simulink model "eVTOL_PX4_2023b"  (R2024b)
settings: Solver=ode4  StartTime=0  StopTime=inf  FixedStep=0.01  RelTol=1e-3
values from neighbouring files (symbols this model uses):
  aDl =     [initdata.mat]
  aDr =     [initdata.mat]
  aDyn =     [initdata.mat]
  Airport = init_airport('PHNL')    [initdata_HIL_eVTOL.m]
  aLat =     [initdata.mat]
  aLon =     [initdata.mat]
  D = Prop.D    [EOM_dt_MC.m]    (also in EOM_get_alf_dt_de_prop_evtol.m = CD * QS)
  dt0 = X(2)    [EOM_get_alf_dt_de_prop_evtol.m]    (also in initdata.mat = 0.258252593971; initdata_HIL_eVTOL.m = EOM_dt_MC)
  EAS0 = TAS0 / EAS2TAS    [initdata_HIL_eVTOL.m]
  FCS = init_FCS    [initdata_HIL_eVTOL.m]
  General = init_layoutdata    [EOM_dt_MC.m]    (also in build_optimized_CA.m; initdata.mat = ; initdata_HIL_eVTOL.m)
  h0 = Con(1)    [EOM_get_alf_dt_de_prop_evtol.m]    (also in initdata.mat = 450; initdata_HIL_eVTOL.m = 50)
  mass = Con(3)    [EOM_get_alf_dt_de_prop_evtol.m]    (also in initdata.mat = 2255.54; initdata_HIL_eVTOL.m = 7)
  Motor = init_motor_evtol    [EOM_dt_MC.m]    (also in initdata.mat = []; initdata_HIL_eVTOL.m)
  Prop = init_propeller_evtol_new    [EOM_dt_MC.m]    (also in initdata_HIL_eVTOL.m)
  R2D = 180/pi    (= 57.2957795131)    [EOM_get_alf_dt_de_prop_evtol.m]    (also in init_FCS.m; init_aerodata_evtol.m; init_airport.m; initdata.mat)
  SAMPLE_TIME = 0.01    [initdata_HIL_eVTOL.m]
  theta0 = -0.0510981441662    [initdata.mat]
undefined symbols (not defined in the file or in its folder): A1, aDa, aDe, aero, asbhl20env, B1, C1, de0, Earth, Environment, INIT_Data, InitData, Kd, Kp, magnitude, Newton, pProp, Raphson, Tc, WGS84
libraries: simulink_extras x63, vrlib x48, sharedtransform x28, simulink x22, slpidlib x20, sharedutil x20, matrix_library x18, aerolibwindfilters x12, aerolibobsolete x8, aerolibasang x8, aerolibatmos2 x6, aerolibfltsims x6
(part 2 of 17)

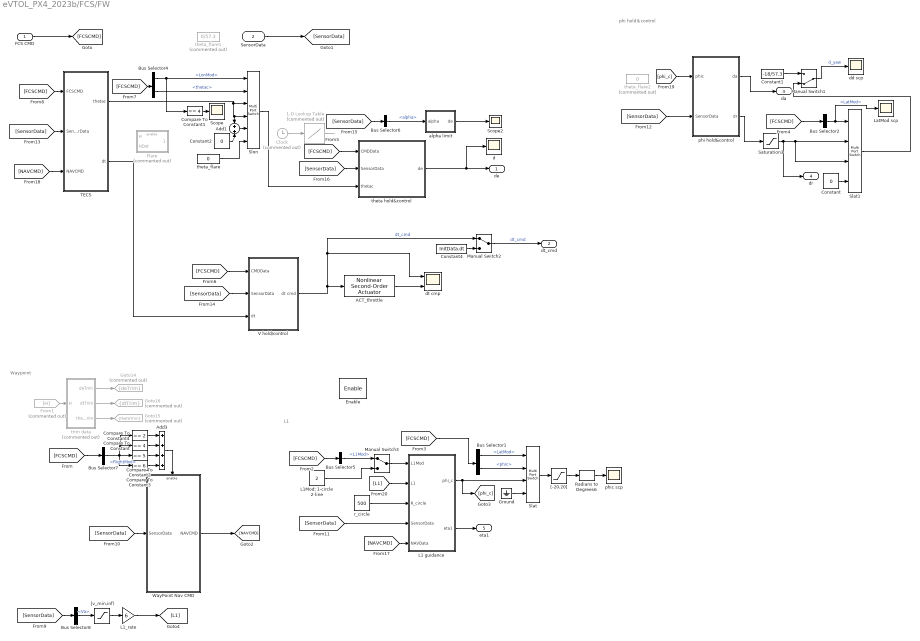
== system eVTOL_PX4_2023b/FCS/FW ==
  note: phi hold＆control
  note: L1
  note: Waypoint
  FCS CMD : Inport
  SensorData : Inport  Port=2
  Enable : EnablePort  StatesWhenEnabling=reset
  1-D Lookup Table : Lookup_n-D  Commented=on  NumberOfTableDimensions=1  BreakpointsForDimension1=[0,4,13,1e3]  Table=[-90,-90,0,0]./57.3  InternalRulePriority=Speed  RndMeth=Simplest
  ACT_throttle : aerolibactuator/Nonlinear Second-Order Actuator  wn_fin=50  z_fin=0.8  fin_max=FCS.dt_max  fin_min=FCS.dt_min  fin_maxrate=FCS.dt_rate  fin_act_0=InitData.dt  fin_act_vel=0
  Add1 : Sum  Inputs=+|+
  Add3 : Sum  Inputs=++++
  Bus Selector1 : BusSelector  OutputSignals=LatMod,phic
  Bus Selector2 : BusSelector  OutputSignals=LatMod
  Bus Selector4 : BusSelector  OutputSignals=LonMod,thetac
  Bus Selector5 : BusSelector  OutputSignals=L1Mod
  Bus Selector6 : BusSelector  OutputSignals=alpha
  Bus Selector7 : BusSelector  OutputSignals=FlightMod
  Bus Selector8 : BusSelector  OutputSignals=Va
  Clock : Clock  Commented=on
  Compare To Constant : simulink/Logic and Bit Operations/Compare To Constant  relop===  const=4  OutDataTypeStr=boolean
  Compare To Constant1 : simulink/Logic and Bit Operations/Compare To Constant  relop===  const=4  OutDataTypeStr=uint8  ZeroCross=off
  Compare To Constant2 : simulink/Logic and Bit Operations/Compare To Constant  relop===  const=5  OutDataTypeStr=boolean
  Compare To Constant3 : simulink/Logic and Bit Operations/Compare To Constant  relop===  const=6  OutDataTypeStr=boolean
  Compare To Constant4 : simulink/Logic and Bit Operations/Compare To Constant  relop===  const=2  OutDataTypeStr=boolean
  Constant : Constant  Value=0
  Constant1 : Constant  Value=-18/57.3
  Constant2 : Constant  Value=0
  Constant4 : Constant  Value=InitData.dt
  Flare : Subsystem  Commented=on
  From1 : From  Commented=on  GotoTag=H
      settings: CloseFcn=tagdialog Close
  Goto14 : Goto  Commented=on  GotoTag=deTrim  TagVisibility=scoped
  Goto15 : Goto  Commented=on  GotoTag=thetaTrim  TagVisibility=scoped
  Goto16 : Goto  Commented=on  GotoTag=dtTrim  TagVisibility=scoped
  Ground : Ground
  L1 guidance : Subsystem
  L1Mod: 1-circle 2-line : Constant  Value=2
  L1_rate : Gain  Gain=6
  LatMod scp : Scope
  Manual Switch1 : ManualSwitch  CurrentSetting=0
  Manual Switch2 : ManualSwitch
  Manual Switch3 : ManualSwitch
  Radians to Degrees6 : simulink_extras/Transformations/Radians to Degrees
  Saturation3 : Saturate  UpperLimit=0.3  LowerLimit=-0.3
  Scope : Scope
  Scope2 : Scope
  Slat : MultiPortSwitch  SaturateOnIntegerOverflow=off  InputSameDT=off
  Slat1 : MultiPortSwitch  SaturateOnIntegerOverflow=off  InputSameDT=off
  Slon : MultiPortSwitch  Inputs=5  SaturateOnIntegerOverflow=off  InputSameDT=off
  TECS : Subsystem
  V hold/control : Subsystem
  WayPoint Nav CMD : Subsystem
  "[-20,20]" : Saturate  UpperLimit=20*pi/180  LowerLimit=-20*pi/180
  "[v_min,inf)" : Saturate  UpperLimit=inf  LowerLimit=FCS.V_min
  alpha limit : Subsystem
  d : Scope
  dd scp : Scope
  dt cmp : Scope  NumInputPorts=2
  phi hold&control : Subsystem
  phic scp : Scope
  r_circle : Constant  Value=500
  theta hold&control : Subsystem
  theta_flare : Constant  Value=0
  theta_flare1 : Constant  Commented=on  Value=0/57.3
  theta_flare2 : Constant  Commented=on  Value=0
  trim data : Subsystem  Commented=on
  de : Outport
  dt_cmd : Outport  Port=2
  da : Outport  Port=3
  dr : Outport  Port=4
  eta1 : Outport  Port=5
  wires:
  Compare To Constant4/1 -> Add3/1
  Bus Selector1/1 -> Slat/1  "<LatMod>"
  trim data/1(deTrim) -> Goto14/1
  WayPoint Nav CMD/1(NAVCMD) -> [NAVCMD]
  L1 guidance/2(eta1) -> eta1/1
  Slat/1 -> "[-20,20]"/1
  "[-20,20]"/1 -> Radians to Degrees6/1
  Add3/1 -> WayPoint Nav CMD/Enable
  r_circle/1 -> L1 guidance/3(R_circle)
  alpha limit/1(de) -> Scope2/1
  Ground/1 -> Slat/4
  V hold/control/1(dt cmd) -> Manual Switch2/1, dt cmp/1, ACT_throttle/1  "dt_cmd"
  L1Mod: 1-circle 2-line/1 -> Manual Switch3/2
  Constant4/1 -> Manual Switch2/2
  trim data/3(thetaTrim) -> Goto15/1
  ACT_throttle/1 -> dt cmp/2
  SensorData/1 -> [SensorData]
  Slat1/1 -> Manual Switch1/2
  Manual Switch1/1 -> dd scp/1  "d_yaw"
  Add1/1 -> Slon/5
  theta_flare/1 -> Slon/6
  Bus Selector2/1 -> LatMod scp/1, Slat1/1  "<LatMod>"
  Bus Selector5/1 -> Manual Switch3/1  "<L1Mod>"
  Bus Selector6/1 -> alpha limit/1(alpha)  "<alpha>"
  Bus Selector7/1 -> Compare To Constant3/1, Compare To Constant4/1, Compare To Constant/1, Compare To Constant2/1  "<FlightMod>"
  "[v_min,inf)"/1 -> L1_rate/1
  Clock/1 -> 1-D Lookup Table/1
  TECS/1(thetac) -> Add1/1, Slon/4, Slon/3
  Saturation3/1 -> dr/1, Slat1/3, Slat1/2
  Slon/1 -> theta hold&control/3(thetac)
  Bus Selector4/1 -> Compare To Constant1/1, Slon/1  "<LonMod>"
  1-D Lookup Table/1 -> ?
  TECS/2(dt) -> V hold/control/3(dt)
  Radians to Degrees6/1 -> phic scp/1
  Bus Selector4/2 -> Slon/2  "<thetac>"
  Bus Selector8/1 -> "[v_min,inf)"/1  "<Va>"
  From1/1 -> trim data/1(H)
  Manual Switch3/1 -> L1 guidance/1(L1Mod)
  phi hold&control/2(dr) -> Saturation3/1
  FCS CMD/1 -> [FCSCMD]
  Compare To Constant2/1 -> Add3/3
  Manual Switch2/1 -> dt_cmd/1  "dt_cmd"
  Constant1/1 -> Manual Switch1/1
  Compare To Constant3/1 -> Add3/4
  trim data/2(dtTrim) -> Goto16/1
  Compare To Constant/1 -> Add3/2
  Bus Selector1/2 -> Slat/2  "<phic>"
  Constant2/1 -> Add1/2
  Constant/1 -> Slat1/4
  Compare To Constant1/1 -> Scope/1
  L1 guidance/1(phi_c) -> [phi_c], Slat/3
  theta hold&control/1(de) -> d/1, de/1
  phi hold&control/1(da) -> da/1
  [FCSCMD] -> Bus Selector7/1
  [FCSCMD] -> Bus Selector5/1
  [FCSCMD] -> Bus Selector1/1
  [FCSCMD] -> Bus Selector2/1
  [FCSCMD] -> theta hold&control/1(CMDData)
  [FCSCMD] -> V hold/control/1(CMDData)
  [FCSCMD] -> Bus Selector4/1
  [FCSCMD] -> TECS/1(FCSCMD)
  [SensorData] -> Bus Selector8/1
  [SensorData] -> WayPoint Nav CMD/1(SensorData)
  [SensorData] -> L1 guidance/4(SensorData)
  [SensorData] -> phi hold&control/2(SensorData)
  [SensorData] -> TECS/2(SensorData)
  [SensorData] -> V hold/control/2(SensorData)
  [SensorData] -> Bus Selector6/1
  [SensorData] -> theta hold&control/2(SensorData)
  [NAVCMD] -> L1 guidance/5(NAVData)
  [NAVCMD] -> TECS/3(NAVCMD)
  [phi_c] -> phi hold&control/1(phic)
  L1_rate/1 -> [L1]
  [L1] -> L1 guidance/2(L1)

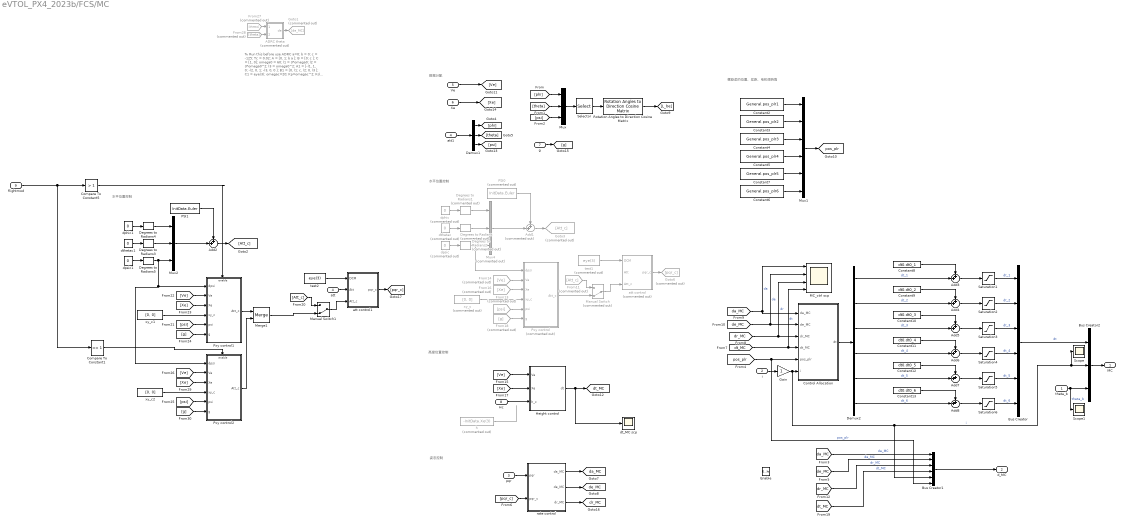
== system eVTOL_PX4_2023b/FCS/MC ==
  note: 数据分配
  note: 螺旋桨的位置、桨距、电机倾转角
  note: 姿态控制
  note: 高度位置控制
  note: 水平位置控制
  note: % Run this before use ADRC
      | a=0;
      | b = 0;
      | c = -125;
      | Tc = 0.02;
      | A = [0, 1; b a ];
      | B = [0; c ];
      | C = [1, 0];
      | omega0 = 60;
      | l1 = 3*omega0;
      | l2 = 3*omega0^2;
      | l3 = omega0^2;
      | A1 = [-l1,  1,  0; -l2,  0,  1; -l3,  0,  0 ];
      | B1 = [0,  l1; c,  l2; 0,  l3 ];
      | C1 = eye(3);
      | omegac=20;
      | Kp=omegac^2;
      | Kd = 2*omegac;
  note: 水平位置控制
  theta_b : Inport
  i : Inport  Port=2
  pqr : Inport  Port=3
  att : Inport  Port=4
  Ve : Inport  Port=5
  Xe : Inport  Port=6
  g : Inport  Port=7
  Hc : Inport  Port=8
  flightmod : Inport  Port=9
  Enable : EnablePort  StatesWhenEnabling=reset
  ADRC theta : Subsystem  Commented=on
  Add1 : Sum  Commented=on  Inputs=++|
  Add{2..8} (7 alike) : Sum  Inputs=++|
  Bus Creator : BusCreator  Inputs=6
  Bus Creator1 : BusCreator  Inputs=6
  Bus Creator2 : BusCreator  Inputs=3
  Compare To Constant1 : simulink/Logic and Bit Operations/Compare To Constant  relop===  const=1  OutDataTypeStr=boolean
  Compare To Constant5 : simulink/Logic and Bit Operations/Compare To Constant  relop=>  const=1  OutDataTypeStr=boolean
  Constant10 : Constant  Value=dt0.dt0_3
  Constant11 : Constant  Value=dt0.dt0_4
  Constant12 : Constant  Value=dt0.dt0_5
  Constant13 : Constant  Value=dt0.dt0_6
  Constant2 : Constant  Value=General.pos_plr1
  Constant3 : Constant  Value=General.pos_plr2
  Constant4 : Constant  Value=General.pos_plr3
  Constant5 : Constant  Value=General.pos_plr4
  Constant6 : Constant  Value=General.pos_plr6
  Constant7 : Constant  Value=General.pos_plr5
  Constant8 : Constant  Value=dt0.dt0_1
  Constant9 : Constant  Value=dt0.dt0_2
  Control Allocation : MATLAB Function  TreatAsAtomicUnit=on
  Degrees to Radians : simulink_extras/Transformations/Degrees to Radians  Commented=on
  Degrees to Radians1 : simulink_extras/Transformations/Degrees to Radians  Commented=on
  Degrees to Radians2 : simulink_extras/Transformations/Degrees to Radians  Commented=on
  Degrees to Radians3 : simulink_extras/Transformations/Degrees to Radians
  Degrees to Radians4 : simulink_extras/Transformations/Degrees to Radians
  Degrees to Radians5 : simulink_extras/Transformations/Degrees to Radians
  Demux1 : Demux  Outputs=3
  Demux2 : Demux  Outputs=6
  From11 : From  Commented=on  GotoTag=Att_c
  From13 : From  Commented=on  GotoTag=psi
  From14 : From  Commented=on  GotoTag=Ve
  From16 : From  Commented=on  GotoTag=Xe
  From18 : From  Commented=on  GotoTag=g
  From27 : From  Commented=on  GotoTag=thetac
  From28 : From  Commented=on  GotoTag=theta
  Gain : Gain
  Goto1 : Goto  Commented=on  GotoTag=de_MC
  Goto3 : Goto  Commented=on  GotoTag=Att_c
  Goto6 : Goto  Commented=on  GotoTag=pqr_c
  Height control : Subsystem
  MC_ctrl scp : Scope  NumInputPorts=4
  Manual Switch : ManualSwitch  Commented=on  CurrentSetting=0
  Manual Switch1 : ManualSwitch  CurrentSetting=0
  Merge1 : Merge
  Mux : Mux  Inputs=3
  Mux1 : Mux  Inputs=6
  Mux2 : Mux  Inputs=3
  Mux4 : Mux  Commented=on  Inputs=3
  PSI0 : Constant  Commented=on  Value=InitData.Euler
  PSI1 : Constant  Value=InitData.Euler
  Pxy control : Subsystem  Commented=on
  Pxy control1 : Subsystem
  Pxy control2 : Subsystem
  Rotation Angles to Direction Cosine Matrix : sharedtransform/Rotation Angles to Direction Cosine Matrix  rotationOrder=ZYX  aMode=aMode
  Saturation{1..6} (6 alike) : Saturate  UpperLimit=1  LowerLimit=0
  Scope : Scope
  Scope1 : Scope
  Selector : Selector  InputPortWidth=3  IndexOptions=Index vector (dialog)  Indices=[3,2,1]  OutputSizes=1
  att control : Subsystem  Commented=on
  att control1 : Subsystem
  att1 : InportShadow  Port=4
  dphic : Constant  Commented=on  Value=0
  dphic1 : Constant  Value=0
  dpsic : Constant  Commented=on  Value=0
  dpsic1 : Constant  Value=0
  dt_MC scp : Scope
  dthetac : Constant  Commented=on  Value=0
  dthetac1 : Constant  Value=0
  h : Constant  Commented=on  Value=-InitData.Xe(3)
  rate control : Subsystem
  test1 : Constant  Commented=on  Value=eye(3)
  test2 : Constant  Value=eye(3)
  xy_c : Constant  Commented=on  Value=[0, 0]
  xy_c1 : Constant  Value=[0, 0]
  xy_c2 : Constant  Value=[0, 0]
  MC : Outport
  d_MC : Outport  Port=2
  tag scope: da_MC=global, de_MC=global, dr_MC=global, dt_MC=global, pos_plr=global
  wires:
  Demux2/3 -> Add5/2  "dt_3"
  Demux2/2 -> Add4/2  "dt_2"
  Demux2/4 -> Add6/2  "dt_4"
  Demux2/1 -> Add3/2  "dt_1"
  Bus Creator/1 -> Bus Creator2/1  "dt"
  Rotation Angles to Direction Cosine Matrix/1 -> [L_be]
  Mux/1 -> Selector/1
  Selector/1 -> Rotation Angles to Direction Cosine Matrix/1
  [phi] -> Mux/1
  [psi] -> Mux/3
  Degrees to Radians/1 -> Mux4/2
  Degrees to Radians2/1 -> Pxy control/1(dpsi), Mux4/3
  [theta] -> Mux/2
  dphic/1 -> Degrees to Radians1/1
  dpsic/1 -> Degrees to Radians2/1
  Degrees to Radians1/1 -> Mux4/1
  [dt_MC] -> MC_ctrl scp/4, Control Allocation/4(dt_MC)  "dt"
  [da_MC] -> MC_ctrl scp/1, Control Allocation/1(da_MC)  "da"
  [de_MC] -> MC_ctrl scp/2, Control Allocation/2(de_MC)  "de"
  [dr_MC] -> MC_ctrl scp/3, Control Allocation/3(dr_MC)  "dr"
  From28/1 -> ADRC theta/2(theta)
  ADRC theta/1(de) -> Goto1/1
  From27/1 -> ADRC theta/1(thetac)
  pqr/1 -> rate control/1(pqr)
  [pqr_c] -> rate control/2(pqr_c)
  ? -> att control/2(Att)
  att control/1(pqr_c) -> Goto6/1
  Mux4/1 -> Add1/2
  From11/1 -> Manual Switch/1
  att1/1 -> Demux1/1
  Demux1/1 -> [phi]
  Demux1/3 -> [psi]
  Demux1/2 -> [theta]
  Ve/1 -> [Ve]
  Xe/1 -> [Xe]
  Pxy control/1(Att_c) -> Manual Switch/2
  xy_c/1 -> Pxy control/4(xy_c)
  Manual Switch/1 -> att control/3(Att_c)
  Add1/1 -> Goto3/1
  PSI0/1 -> Add1/1
  Control Allocation/1(dt) -> Demux2/1
  Height control/1(dt) -> dt_MC scp/1, [dt_MC]
  test1/1 -> att control/1(DCM)
  Hc/1 -> Height control/3(h_c)
  h/1 -> ?
  dthetac/1 -> Degrees to Radians/1
  Demux2/5 -> Add7/2  "dt_5"
  Demux2/6 -> Add8/2  "dt_6"
  rate control/1(da_MC) -> [da_MC]
  rate control/2(de_MC) -> [de_MC]
  rate control/3(dr_MC) -> [dr_MC]
  Constant2/1 -> Mux1/1
  Constant3/1 -> Mux1/2
  Constant4/1 -> Mux1/3
  Constant5/1 -> Mux1/4
  Constant7/1 -> Mux1/5
  Constant6/1 -> Mux1/6
  Mux1/1 -> [pos_plr]
  [pos_plr] -> Bus Creator1/6, Control Allocation/5(pos_plr)  "pos_plr"
  Gain/1 -> Bus Creator1/5, Scope/1, Bus Creator2/2, Control Allocation/6(i)  "i"
  theta_b/1 -> Scope1/1, Bus Creator2/3  "theta_b"
  Bus Creator2/1 -> MC/1
  Saturation1/1 -> Bus Creator/1  "dt_1"
  Saturation2/1 -> Bus Creator/2  "dt_2"
  Saturation3/1 -> Bus Creator/3  "dt_3"
  Saturation4/1 -> Bus Creator/4  "dt_4"
  Saturation5/1 -> Bus Creator/5  "dt_5"
  Saturation6/1 -> Bus Creator/6  "dt_6"
  Constant8/1 -> Add3/1
  Add3/1 -> Saturation1/1
  Constant9/1 -> Add4/1
  Add4/1 -> Saturation2/1
  Constant10/1 -> Add5/1
  Add5/1 -> Saturation3/1
  Constant11/1 -> Add6/1
  Add6/1 -> Saturation4/1
  Constant12/1 -> Add7/1
  Add7/1 -> Saturation5/1
  Constant13/1 -> Add8/1
  Add8/1 -> Saturation6/1
  From13/1 -> Pxy control/5(psi)
  From14/1 -> Pxy control/2(Ve)
  [Ve] -> Height control/1(Ve)
  From16/1 -> Pxy control/3(Xe)
  [Xe] -> Height control/2(Xe)
  g/1 -> [g]
  From18/1 -> Pxy control/6(g)
  i/1 -> Gain/1
  [da_MC] -> Bus Creator1/1  "da_MC"
  [de_MC] -> Bus Creator1/2  "de_MC"
  [dr_MC] -> Bus Creator1/3  "dr_MC"
  [dt_MC] -> Bus Creator1/4  "dt_MC"
  Bus Creator1/1 -> d_MC/1
  dphic1/1 -> Degrees to Radians4/1
  PSI1/1 -> Add2/1
  Degrees to Radians3/1 -> Mux2/2
  [g] -> Pxy control1/6(g)
  Pxy control1/1(Att_c) -> Merge1/1
  [Att_c] -> Manual Switch1/1
  dthetac1/1 -> Degrees to Radians3/1
  xy_c1/1 -> Pxy control1/4(xy_c)
  Mux2/1 -> Add2/2
  test2/1 -> att control1/1(DCM)
  Degrees to Radians4/1 -> Mux2/1
  [psi] -> Pxy control1/5(psi)
  Manual Switch1/1 -> att control1/3(Att_c)
  Add2/1 -> [Att_c]
  att/1 -> att control1/2(Att)
  [Ve] -> Pxy control1/2(Ve)
  [Xe] -> Pxy control1/3(Xe)
  dpsic1/1 -> Degrees to Radians5/1
  att control1/1(pqr_c) -> [pqr_c]
  Compare To Constant5/1 -> Pxy control1/Enable
  Degrees to Radians5/1 -> Pxy control2/1(dpsi), Pxy control1/1(dpsi), Mux2/3
  [Ve] -> Pxy control2/2(Ve)
  [psi] -> Pxy control2/5(psi)
  [Xe] -> Pxy control2/3(Xe)
  Pxy control2/1(Att_c) -> Merge1/2
  xy_c2/1 -> Pxy control2/4(xy_c)
  [g] -> Pxy control2/6(g)
  Compare To Constant1/1 -> Pxy control2/Enable
  Merge1/1 -> Manual Switch1/2
  flightmod/1 -> Compare To Constant1/1, Compare To Constant5/1

== system eVTOL_PX4_2023b/FCS/control selector ==
  note: CtrlMod:
      | 1-pqr control
      | 2-att control
      | 3-path angle control
      | 4-way point control
      | 5-TakeOff
      | 6-Parachute land
  note: FlightStage
      | 1-Ready
      | 2-TakeOff
      | 3-PullUp
      | 4-Climb
      | 5-Cruise, 5.1-circle, 5.2-line
      | 6-Return
      | 7-Approach
      | 8-Flare
      | 9-TouchDown
      | 10-Taxi
      | 11-GoAround
      | 12-Parachute
  Bus Selector1 : BusSelector  Commented=on  OutputSignals=FlightMod
  Constant1 : Constant  Commented=on
  Constant8 : Constant  Commented=on  Value=0
  Constant9 : Constant  Commented=on
  From1 : From  Commented=on  GotoTag=CutAct
  From2 : From  Commented=on  GotoTag=CutAct
  From3 : From  Commented=on  GotoTag=CutAct
  From9 : From  Commented=on  GotoTag=deTrim  TagVisibility=scoped
      settings: CloseFcn=tagdialog Close
  Goto5 : Goto  Commented=on  GotoTag=CutAct
  Merge : Merge  Commented=on
  Product{,1..3} (4 alike) : Product  Commented=on
  Radians to Degrees1 : simulink_extras/Transformations/Radians to Degrees  Commented=on
  Scope : Scope  Commented=on
  Scope1 : Scope  Commented=on
  Switch Case : SwitchCase  Commented=on  CaseConditions={[2,12]}
  Switch Case Action Subsystem1 : Subsystem  Commented=on  TreatAsAtomicUnit=on
  Switch Case Action Subsystem2 : Subsystem  Commented=on  TreatAsAtomicUnit=on
  dr scp : Scope  Commented=on
  dt scp : Scope  Commented=on
  wires:
  Product/1 -> dt scp/1
  Switch Case Action Subsystem2/1(Out1) -> Merge/1
  Constant9/1 -> Switch Case Action Subsystem1/1(In1)  "keep"
  Switch Case Action Subsystem1/1(Out1) -> Merge/2
  Switch Case/1 -> Switch Case Action Subsystem2/Action
  Bus Selector1/1 -> Scope1/1, Switch Case/1  "<FlightMod>"
  Switch Case/2 -> Switch Case Action Subsystem1/Action
  Constant8/1 -> Switch Case Action Subsystem2/1(In1)  "cut"
  Merge/1 -> Goto5/1
  Constant1/1 -> Product/1
  From1/1 -> Product1/2
  From3/1 -> Product3/2
  From2/1 -> Product2/2
  Product2/1 -> dr scp/1
  Product1/1 -> Radians to Degrees1/1
  Radians to Degrees1/1 -> Scope/1
  ? -> ?

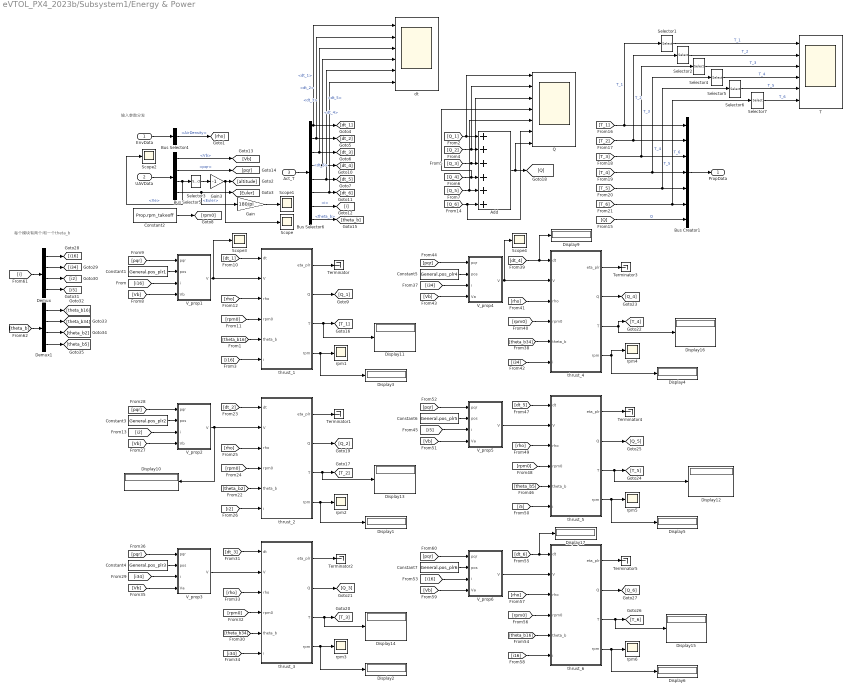
== system eVTOL_PX4_2023b/Subsystem1/Energy & Power ==
  note: 每个模块有两个i和一个theta_b
  note: 输入参数分发
  EnvData : Inport
  UAVData : Inport  Port=2
  Act_T : Inport  Port=3
  Add : Sum  Inputs=++++++
  Bus Creator1 : BusCreator  Inputs=7
  Bus Selector4 : BusSelector  OutputSignals=AirDensity
  Bus Selector5 : BusSelector  OutputSignals=Vb,pqr,Xe,Euler
  Bus Selector6 : BusSelector  OutputSignals=dt_1,dt_2,dt_3,dt_4,dt_5,dt_6,i,theta_b
  Constant1 : Constant  Value=General.pos_plr1
  Constant2 : Constant  Value=Prop.rpm_takeoff
  Constant3 : Constant  Value=General.pos_plr2
  Constant4 : Constant  Value=General.pos_plr3
  Constant5 : Constant  Value=General.pos_plr4
  Constant6 : Constant  Value=General.pos_plr5
  Constant7 : Constant  Value=General.pos_plr6
  Demux : Demux
  Demux1 : Demux
  Display{1..6,9..17} (15 alike) : Display
  Gain : Gain  Gain=180/pi
  Gain3 : Gain  Gain=-1
  Q : Scope  NumInputPorts=7
  Scope{,1..4} (5 alike) : Scope
  Selector{1..7} (7 alike) : Selector  InputPortWidth=3  IndexOptions=Index vector (dialog)  Indices=3  OutputSizes=1
  T : Scope  NumInputPorts=6
  Terminator{,1..5} (6 alike) : Terminator
  V_prop1 : Subsystem
  V_prop2 : Subsystem
  V_prop3 : Subsystem
  V_prop4 : Subsystem
  V_prop5 : Subsystem
  V_prop6 : Subsystem
  dt : Scope  NumInputPorts=6
  rpm{1..6} (6 alike) : Scope
  thrust_1 : Subsystem
  thrust_2 : Subsystem
  thrust_3 : Subsystem
  thrust_4 : Subsystem
  thrust_5 : Subsystem
  thrust_6 : Subsystem
  PropData : Outport  VectorParamsAs1DForOutWhenUnconnected=off
  wires:
  Act_T/1 -> Bus Selector6/1
  [dt_1] -> thrust_1/1(dt)
  thrust_1/4(rpm) -> Display3/1, rpm1/1
  Constant1/1 -> V_prop1/2(pos)
  [rho] -> thrust_1/3(rho)
  [rpm0] -> thrust_1/4(rpm0)
  thrust_1/1(eta_plr) -> Terminator/1
  [pqr] -> V_prop1/1(pqr)
  [Vb] -> V_prop1/4(Vb)
  EnvData/1 -> Bus Selector4/1
  Bus Selector4/1 -> [rho]  "<AirDensity>"
  Bus Selector5/2 -> [pqr]  "<pqr>"
  Selector3/1 -> Gain3/1
  UAVData/1 -> Bus Selector5/1
  Bus Selector5/4 -> Gain/1, [Euler]  "<Euler>"
  Bus Selector5/1 -> [Vb]  "<Vb>"
  Bus Selector5/3 -> Scope2/1, Selector3/1  "<Xe>"
  Bus Selector6/1 -> dt/1, [dt_1]  "<dt_1>"
  Bus Selector6/5 -> dt/5, [dt_5]  "<dt_5>"
  Bus Selector6/3 -> dt/3, [dt_3]  "<dt_3>"
  Bus Selector6/2 -> [dt_2], dt/2  "<dt_2>"
  V_prop1/1(V) -> Scope3/1, thrust_1/2(V)
  [i16] -> V_prop1/3(i)
  Constant2/1 -> [rpm0]
  [theta_b16] -> thrust_1/5(theta_b)
  thrust_1/2(Q) -> [Q_1]
  Bus Selector6/4 -> dt/4, [dt_4]  "<dt_4>"
  Bus Selector6/6 -> dt/6, [dt_6]  "<dt_6>"
  Bus Selector6/7 -> [i]  "<i>"
  Bus Selector6/8 -> [theta_b]  "<theta_b>"
  [i16] -> thrust_1/6(i)
  thrust_1/3(T) -> Display11/1, [T_1]
  [Q_1] -> Q/1, Add/1
  [Q_6] -> Q/6, Add/6
  [Q_5] -> Q/5, Add/5
  [Q_4] -> Q/4, Add/4
  [Q_3] -> Q/3, Add/3
  [Q_2] -> Q/2, Add/2
  Add/1 -> Q/7, [Q]
  [Q] -> Bus Creator1/7  "Q"
  [T_1] -> Selector1/1, Bus Creator1/1  "T_1"
  [T_2] -> Selector2/1, Bus Creator1/2  "T_2"
  [T_3] -> Bus Creator1/3, Selector4/1  "T_3"
  [T_4] -> Bus Creator1/4, Selector5/1  "T_4"
  [T_5] -> Bus Creator1/5, Selector6/1  "T_5"
  [T_6] -> Bus Creator1/6, Selector7/1  "T_6"
  Bus Creator1/1 -> PropData/1
  [theta_b2] -> thrust_2/5(theta_b)
  Constant3/1 -> V_prop2/2(pos)
  [dt_2] -> thrust_2/1(dt)
  V_prop2/1(V) -> Display10/1, thrust_2/2(V)
  thrust_2/2(Q) -> [Q_2]
  thrust_2/1(eta_plr) -> Terminator1/1
  [i2] -> V_prop2/3(i)
  thrust_2/3(T) -> [T_2], Display13/1
  [rpm0] -> thrust_2/4(rpm0)
  [Vb] -> V_prop2/4(Vb)
  [pqr] -> V_prop2/1(pqr)
  [i2] -> thrust_2/6(i)
  thrust_2/4(rpm) -> rpm2/1, Display1/1
  [rho] -> thrust_2/3(rho)
  [rho] -> thrust_3/3(rho)
  [pqr] -> V_prop3/1(pqr)
  [Vb] -> V_prop3/4(Va)
  [i34] -> V_prop3/3(i)
  thrust_3/2(Q) -> [Q_3]
  V_prop3/1(V) -> thrust_3/2(V)
  [rpm0] -> thrust_3/4(rpm0)
  [dt_3] -> thrust_3/1(dt)
  thrust_3/4(rpm) -> Display2/1, rpm3/1
  [theta_b34] -> thrust_3/5(theta_b)
  Constant4/1 -> V_prop3/2(pos)
  thrust_3/1(eta_plr) -> Terminator2/1
  [i34] -> thrust_3/6(i)
  thrust_3/3(T) -> Display14/1, [T_3]
  [i34] -> thrust_4/6(i)
  [theta_b34] -> thrust_4/5(theta_b)
  Constant5/1 -> V_prop4/2(pos)
  thrust_4/1(eta_plr) -> Terminator3/1
  thrust_4/3(T) -> [T_4], Display16/1
  [dt_4] -> Display9/1, thrust_4/1(dt)
  V_prop4/1(V) -> Scope4/1, thrust_4/2(V)
  [rpm0] -> thrust_4/4(rpm0)
  [i34] -> V_prop4/3(i)
  thrust_4/4(rpm) -> rpm4/1, Display4/1
  [Vb] -> V_prop4/4(Va)
  [pqr] -> V_prop4/1(pqr)
  [rho] -> thrust_4/3(rho)
  thrust_4/2(Q) -> [Q_4]
  thrust_5/2(Q) -> [Q_5]
  thrust_5/3(T) -> Display12/1, [T_5]
  [rho] -> thrust_5/3(rho)
  [pqr] -> V_prop5/1(pqr)
  [rpm0] -> thrust_5/4(rpm0)
  Constant6/1 -> V_prop5/2(pos)
  thrust_5/1(eta_plr) -> Terminator4/1
  [dt_5] -> thrust_5/1(dt)
  thrust_5/4(rpm) -> Display5/1, rpm5/1
  [i5] -> V_prop5/3(i)
  V_prop5/1(V) -> thrust_5/2(V)
  [i5] -> thrust_5/6(i)
  [theta_b5] -> thrust_5/5(theta_b)
  [Vb] -> V_prop5/4(Va)
  [i16] -> V_prop6/3(i)
  [Vb] -> V_prop6/4(Va)
  thrust_6/1(eta_plr) -> Terminator5/1
  V_prop6/1(V) -> thrust_6/2(V)
  [dt_6] -> Display17/1, thrust_6/1(dt)
  [theta_b16] -> thrust_6/5(theta_b)
  thrust_6/2(Q) -> [Q_6]
  thrust_6/3(T) -> Display15/1, [T_6]
  Constant7/1 -> V_prop6/2(pos)
  [rho] -> thrust_6/3(rho)
  thrust_6/4(rpm) -> Display6/1, rpm6/1
  [pqr] -> V_prop6/1(pqr)
  [rpm0] -> thrust_6/4(rpm0)
  [i16] -> thrust_6/6(i)
  Selector1/1 -> T/1  "T_1"
  Selector2/1 -> T/2  "T_2"
  Selector4/1 -> T/3  "T_3"
  Selector5/1 -> T/4  "T_4"
  Selector6/1 -> T/5  "T_5"
  Selector7/1 -> T/6  "T_6"
  Gain3/1 -> Scope/1, [altitude]
  Gain/1 -> Scope1/1
  [i] -> Demux/1
  Demux/1 -> [i16]
  Demux/2 -> [i34]
  Demux/3 -> [i2]
  Demux/4 -> [i5]
  Demux1/2 -> [theta_b34]
  Demux1/3 -> [theta_b2]
  Demux1/1 -> [theta_b16]
  [theta_b] -> Demux1/1
  Demux1/4 -> [theta_b5]

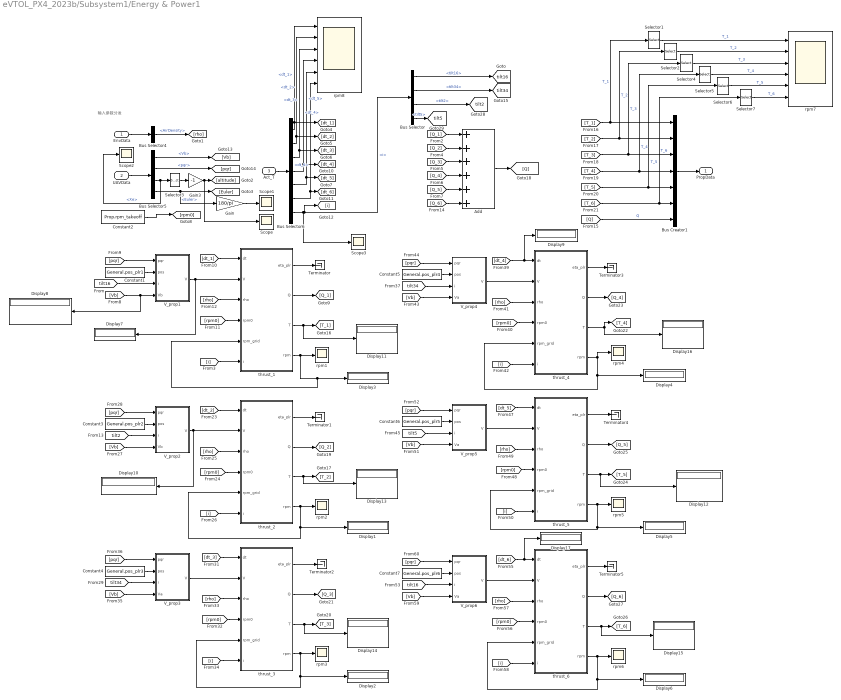
== system eVTOL_PX4_2023b/Subsystem1/Energy & Power1 ==
  note: 输入参数分发
  EnvData : Inport
  UAVData : Inport  Port=2
  Act_T : Inport  Port=3
  Add : Sum  Inputs=++++++
  Bus Creator1 : BusCreator  Inputs=7
  Bus Selector : BusSelector  OutputSignals=tilt16,tilt34,tilt2,tilt5
  Bus Selector4 : BusSelector  OutputSignals=AirDensity
  Bus Selector5 : BusSelector  OutputSignals=Vb,pqr,Xe,Euler
  Bus Selector6 : BusSelector  OutputSignals=dt_1,dt_2,dt_3,dt_4,dt_5,dt_6,i
  Constant1 : Constant  Value=General.pos_plr1
  Constant2 : Constant  Value=Prop.rpm_takeoff
  Constant3 : Constant  Value=General.pos_plr2
  Constant4 : Constant  Value=General.pos_plr3
  Constant5 : Constant  Value=General.pos_plr4
  Constant6 : Constant  Value=General.pos_plr5
  Constant7 : Constant  Value=General.pos_plr6
  Display{1..17} (17 alike) : Display
  Gain : Gain  Gain=180/pi
  Gain3 : Gain  Gain=-1
  Scope{,1..3} (4 alike) : Scope
  Selector{1..7} (7 alike) : Selector  InputPortWidth=3  IndexOptions=Index vector (dialog)  Indices=3  OutputSizes=1
  Terminator{,1..5} (6 alike) : Terminator
  V_prop1 : Subsystem
  V_prop2 : Subsystem
  V_prop3 : Subsystem
  V_prop4 : Subsystem
  V_prop5 : Subsystem
  V_prop6 : Subsystem
  rpm{1..6} (6 alike) : Scope
  rpm7 : Scope  NumInputPorts=6
  rpm8 : Scope  NumInputPorts=6
  thrust_1 : Subsystem
  thrust_2 : Subsystem
  thrust_3 : Subsystem
  thrust_4 : Subsystem
  thrust_5 : Subsystem
  thrust_6 : Subsystem
  PropData : Outport  VectorParamsAs1DForOutWhenUnconnected=off
  tag scope: tilt16=global, tilt2=global, tilt34=global, tilt5=global
  wires:
  Act_T/1 -> Bus Selector6/1
  [dt_1] -> thrust_1/1(dt)
  Constant1/1 -> V_prop1/2(pos)
  [rho] -> thrust_1/3(rho)
  [rpm0] -> thrust_1/4(rpm0)
  thrust_1/1(eta_plr) -> Terminator/1
  [pqr] -> V_prop1/1(pqr)
  [Vb] -> Display8/1, V_prop1/4(Vb)
  EnvData/1 -> Bus Selector4/1
  Bus Selector4/1 -> [rho]  "<AirDensity>"
  Bus Selector5/2 -> [pqr]  "<pqr>"
  Selector3/1 -> Gain3/1
  UAVData/1 -> Bus Selector5/1
  Bus Selector5/4 -> Gain/1, [Euler]  "<Euler>"
  Bus Selector5/1 -> [Vb]  "<Vb>"
  Bus Selector5/3 -> Scope2/1, Selector3/1  "<Xe>"
  Bus Selector6/1 -> rpm8/1, [dt_1]  "<dt_1>"
  Bus Selector6/5 -> [dt_5], rpm8/5  "<dt_5>"
  Bus Selector6/3 -> [dt_3], rpm8/3  "<dt_3>"
  Bus Selector6/2 -> [dt_2], rpm8/2  "<dt_2>"
  V_prop1/1(V) -> thrust_1/2(V), Display7/1
  [tilt16] -> V_prop1/3(i)
  Constant2/1 -> [rpm0]
  thrust_1/4(rpm) -> thrust_1/5(rpm_grid), Display3/1, rpm1/1
  thrust_1/2(Q) -> [Q_1]
  Bus Selector6/4 -> [dt_4], rpm8/4  "<dt_4>"
  Bus Selector6/6 -> rpm8/6, [dt_6]  "<dt_6>"
  Bus Selector6/7 -> Scope3/1, Bus Selector/1, [i]  "<i>"
  [i] -> thrust_1/6(i)
  thrust_1/3(T) -> Display11/1, [T_1]
  [Q_1] -> Add/1
  [Q_6] -> Add/6
  [Q_5] -> Add/5
  [Q_4] -> Add/4
  [Q_3] -> Add/3
  [Q_2] -> Add/2
  Add/1 -> [Q]
  [Q] -> Bus Creator1/7  "Q"
  [T_1] -> Selector1/1, Bus Creator1/1  "T_1"
  [T_2] -> Selector2/1, Bus Creator1/2  "T_2"
  [T_3] -> Bus Creator1/3, Selector4/1  "T_3"
  [T_4] -> Bus Creator1/4, Selector5/1  "T_4"
  [T_5] -> Bus Creator1/5, Selector6/1  "T_5"
  [T_6] -> Bus Creator1/6, Selector7/1  "T_6"
  Bus Creator1/1 -> PropData/1
  thrust_2/4(rpm) -> rpm2/1, thrust_2/5(rpm_grid), Display1/1
  Constant3/1 -> V_prop2/2(pos)
  [dt_2] -> thrust_2/1(dt)
  V_prop2/1(V) -> Display10/1, thrust_2/2(V)
  thrust_2/2(Q) -> [Q_2]
  thrust_2/1(eta_plr) -> Terminator1/1
  [tilt2] -> V_prop2/3(i)
  thrust_2/3(T) -> [T_2], Display13/1
  [rpm0] -> thrust_2/4(rpm0)
  [Vb] -> V_prop2/4(Vb)
  [pqr] -> V_prop2/1(pqr)
  [i] -> thrust_2/6(i)
  [rho] -> thrust_2/3(rho)
  [rho] -> thrust_3/3(rho)
  [pqr] -> V_prop3/1(pqr)
  [Vb] -> V_prop3/4(Va)
  [tilt34] -> V_prop3/3(i)
  thrust_3/2(Q) -> [Q_3]
  V_prop3/1(V) -> thrust_3/2(V)
  [rpm0] -> thrust_3/4(rpm0)
  [dt_3] -> thrust_3/1(dt)
  thrust_3/4(rpm) -> thrust_3/5(rpm_grid), Display2/1, rpm3/1
  Constant4/1 -> V_prop3/2(pos)
  thrust_3/1(eta_plr) -> Terminator2/1
  [i] -> thrust_3/6(i)
  thrust_3/3(T) -> Display14/1, [T_3]
  [i] -> thrust_4/6(i)
  thrust_4/4(rpm) -> rpm4/1, thrust_4/5(rpm_grid), Display4/1
  Constant5/1 -> V_prop4/2(pos)
  thrust_4/1(eta_plr) -> Terminator3/1
  thrust_4/3(T) -> [T_4], Display16/1
  [dt_4] -> Display9/1, thrust_4/1(dt)
  V_prop4/1(V) -> thrust_4/2(V)
  [rpm0] -> thrust_4/4(rpm0)
  [tilt34] -> V_prop4/3(i)
  [Vb] -> V_prop4/4(Va)
  [pqr] -> V_prop4/1(pqr)
  [rho] -> thrust_4/3(rho)
  thrust_4/2(Q) -> [Q_4]
  thrust_5/2(Q) -> [Q_5]
  thrust_5/3(T) -> Display12/1, [T_5]
  [rho] -> thrust_5/3(rho)
  [pqr] -> V_prop5/1(pqr)
  [rpm0] -> thrust_5/4(rpm0)
  Constant6/1 -> V_prop5/2(pos)
  thrust_5/1(eta_plr) -> Terminator4/1
  [dt_5] -> thrust_5/1(dt)
  [tilt5] -> V_prop5/3(i)
  V_prop5/1(V) -> thrust_5/2(V)
  [i] -> thrust_5/6(i)
  thrust_5/4(rpm) -> thrust_5/5(rpm_grid), Display5/1, rpm5/1
  [Vb] -> V_prop5/4(Va)
  [tilt16] -> V_prop6/3(i)
  [Vb] -> V_prop6/4(Va)
  thrust_6/1(eta_plr) -> Terminator5/1
  V_prop6/1(V) -> thrust_6/2(V)
  [dt_6] -> Display17/1, thrust_6/1(dt)
  thrust_6/4(rpm) -> thrust_6/5(rpm_grid), Display6/1, rpm6/1
  thrust_6/2(Q) -> [Q_6]
  thrust_6/3(T) -> Display15/1, [T_6]
  Constant7/1 -> V_prop6/2(pos)
  [rho] -> thrust_6/3(rho)
  [pqr] -> V_prop6/1(pqr)
  [rpm0] -> thrust_6/4(rpm0)
  [i] -> thrust_6/6(i)
  Selector1/1 -> rpm7/1  "T_1"
  Selector2/1 -> rpm7/2  "T_2"
  Selector4/1 -> rpm7/3  "T_3"
  Selector5/1 -> rpm7/4  "T_4"
  Selector6/1 -> rpm7/5  "T_5"
  Selector7/1 -> rpm7/6  "T_6"
  Gain3/1 -> Scope/1, [altitude]
  Gain/1 -> Scope1/1
  Bus Selector/1 -> [tilt16]  "<tilt16>"
  Bus Selector/2 -> [tilt34]  "<tilt34>"
  Bus Selector/3 -> [tilt2]  "<tilt2>"
  Bus Selector/4 -> [tilt5]  "<tilt5>"

== system eVTOL_PX4_2023b/Subsystem1/Environment ==
  plane : Inport
  Bus Creator : BusCreator  Inputs=8
  Bus Selector : BusSelector  OutputSignals=Xe,Ve,DCM_be
  COESA Atmosphere Model : aerolibatmos2/COESA Atmosphere Model  units=Metric (MKS)  spec=1976 COESA-extended U.S. Standard Atmosphere  model=Profile  profile_var=High temperature  profile_percent=1%  profile_alt=5 km (16404 ft)  envelope_var=High temperature  envelope_percent=1%  action=Warning
  Height : Selector  InputPortWidth=3  IndexOptions=Index vector (dialog)  Indices=[3]  OutputSizes=1
  Latitude : Constant  Value=40
  Terrain : Subsystem
  WGS84 Gravity Model : aerolibobsolete/WGS84 Gravity Model  model=WGS84 Taylor Series  units=Metric (MKS)  no_atmos=on  precessing=on  month=February  day=1  year=2000  no_centrifugal=on  action=None
  Wind Models : Subsystem
  x : Selector  InputPortWidth=3  IndexOptions=Index vector (dialog)  Indices=1  OutputSizes=1
  z-->h : Abs
  Envm : Outport  InitialOutput=0  VectorParamsAs1DForOutWhenUnconnected=off
  wires:
  COESA Atmosphere Model/4 -> Bus Creator/7  "AirDensity"
  COESA Atmosphere Model/2 -> Bus Creator/5  "a"
  COESA Atmosphere Model/3 -> Bus Creator/6  "Po"
  COESA Atmosphere Model/1 -> Bus Creator/4  "To"
  Height/1 -> z-->h/1
  Bus Creator/1 -> Envm/1  "EnvmData"
  plane/1 -> Bus Selector/1
  z-->h/1 -> COESA Atmosphere Model/1, WGS84 Gravity Model/1, Wind Models/3(Altitude)
  Bus Selector/1 -> x/1, Terrain/1(Xe), Height/1  "<Xe>"
  Bus Selector/2 -> Wind Models/2(Ve)  "<Ve>"
  Bus Selector/3 -> Wind Models/4(DCM)  "<DCM_be>"
  Latitude/1 -> WGS84 Gravity Model/2
  WGS84 Gravity Model/1 -> Bus Creator/8  "g"
  Terrain/1(hground) -> Bus Creator/1  "hground"
  Wind Models/1(ug,vg,wg1) -> Bus Creator/2
  Wind Models/2(pg,qg,rg1) -> Bus Creator/3
  x/1 -> Wind Models/1(Xe_x)

== system eVTOL_PX4_2023b/Subsystem1/Environment1 ==
  plane : Inport
  Bus Creator : BusCreator  Inputs=8
  Bus Selector : BusSelector  OutputSignals=Xe,Ve,DCM_be
  COESA Atmosphere Model : aerolibatmos2/COESA Atmosphere Model  units=Metric (MKS)  spec=1976 COESA-extended U.S. Standard Atmosphere  model=Profile  profile_var=High temperature  profile_percent=1%  profile_alt=5 km (16404 ft)  envelope_var=High temperature  envelope_percent=1%  action=Warning
  Height : Selector  InputPortWidth=3  IndexOptions=Index vector (dialog)  Indices=[3]  OutputSizes=1
  Latitude : Constant  Value=40
  Terrain : Subsystem
  WGS84 Gravity Model : aerolibobsolete/WGS84 Gravity Model  model=WGS84 Taylor Series  units=Metric (MKS)  no_atmos=on  precessing=on  month=February  day=1  year=2000  no_centrifugal=on  action=None
  Wind Models : Subsystem
  x : Selector  InputPortWidth=3  IndexOptions=Index vector (dialog)  Indices=1  OutputSizes=1
  z-->h : Abs
  Envm : Outport  InitialOutput=0  VectorParamsAs1DForOutWhenUnconnected=off
  wires:
  COESA Atmosphere Model/4 -> Bus Creator/7  "AirDensity"
  COESA Atmosphere Model/2 -> Bus Creator/5  "a"
  COESA Atmosphere Model/3 -> Bus Creator/6  "Po"
  COESA Atmosphere Model/1 -> Bus Creator/4  "To"
  Height/1 -> z-->h/1
  Bus Creator/1 -> Envm/1  "EnvmData"
  plane/1 -> Bus Selector/1
  z-->h/1 -> COESA Atmosphere Model/1, WGS84 Gravity Model/1, Wind Models/3(Altitude)
  Bus Selector/1 -> x/1, Terrain/1(Xe), Height/1  "<Xe>"
  Bus Selector/2 -> Wind Models/2(Ve)  "<Ve>"
  Bus Selector/3 -> Wind Models/4(DCM)  "<DCM_be>"
  Latitude/1 -> WGS84 Gravity Model/2
  WGS84 Gravity Model/1 -> Bus Creator/8  "g"
  Terrain/1(hground) -> Bus Creator/1  "hground"
  Wind Models/1(ug,vg,wg1) -> Bus Creator/2
  Wind Models/2(pg,qg,rg1) -> Bus Creator/3
  x/1 -> Wind Models/1(Xe_x)

== system eVTOL_PX4_2023b/Subsystem1/airframe ==
  note: 只进行纵向[1,0,1][0,1,0]
      | 进行纵向+横向[1,1,1][1,1,0]
      | 进行纵向+航向[1,0,1][0,1,1]
  EnvmData : Inport
  prop : Inport  Port=2
  Act_surface : Inport  Port=3
  SW : Inport  Port=4
  6DoF (Euler Angles)1 : aerolibobsolete/6DoF (Euler Angles)  units=Metric (MKS)  mtype=Fixed  rep=Euler Angles  xme_0=InitData.Xe  Vm_0=InitData.Vb  eul_0=InitData.Euler+[0,0,0]/57.3  pm_0=InitData.pqr  mass_0=InitData.mass0  mass_e=0.5  mass_f=2.0  inertia=Mass.Inertial  inertia_e=eye(3)  inertia_f=2*eye(3)  k_quat=1.0
  Bus Creator : BusCreator  Inputs=25
  Constant3 : Constant  Value=mass
  Flight Conditions : Subsystem  AncestorBlock=asbhl20vehicle/Vehicle/Aerodynamic/DerivedConditions
      settings: LibrarySourceBlock=asbhl20vehicle/Vehicle/Aerodynamic/DerivedConditions
  Fly : Constant
  Gain : Gain  Gain=[1,1,1]
  Gain1 : Gain  Gain=[1,1,1]
  Product : Product
  Product1 : Product
  Switch2 : Switch  Criteria=u2 > Threshold  SaturateOnIntegerOverflow=off  InputSameDT=off
  force moment : Subsystem
  init : Constant  Value=0
  UAVData : Outport  VectorParamsAs1DForOutWhenUnconnected=off
  wires:
  prop/1 -> force moment/3(prop)
  6DoF (Euler Angles)1/1 -> Bus Creator/1  "Ve"
  6DoF (Euler Angles)1/2 -> Bus Creator/2  "Xe"
  6DoF (Euler Angles)1/8 -> Bus Creator/8  "Ab"
  6DoF (Euler Angles)1/7 -> Bus Creator/7  "pqr_dot"
  6DoF (Euler Angles)1/6 -> Bus Creator/6  "pqr"
  6DoF (Euler Angles)1/5 -> Bus Creator/5  "Vb"
  Act_surface/1 -> force moment/2(Act_surface)
  Bus Creator/1 -> UAVData/1, force moment/1(PlantData), Flight Conditions/2(PlantData)  "UAVData"
  EnvmData/1 -> Flight Conditions/1(EnvmData), force moment/4(EnvmData)
  Flight Conditions/6(Beta) -> Bus Creator/14  "beta"
  Flight Conditions/7(V) -> Bus Creator/15  "Va"
  Flight Conditions/9(pqrWind) -> Bus Creator/17  "pqrWind"
  Flight Conditions/10(Mach) -> Bus Creator/18  "mach"
  Flight Conditions/11(Qbar) -> Bus Creator/19  "Q"
  Flight Conditions/12(gamma) -> Bus Creator/20  "gamma"
  Flight Conditions/5(AlphaDot) -> Bus Creator/13  "alphaDot"
  6DoF (Euler Angles)1/4 -> Bus Creator/4  "DCM_be"
  Constant3/1 -> Bus Creator/25  "mass"
  Flight Conditions/13(chi) -> Bus Creator/21  "chi"
  Flight Conditions/14(Po) -> Bus Creator/22  "Po"
  Flight Conditions/15(To) -> Bus Creator/23  "To"
  Flight Conditions/16(g) -> Bus Creator/24  "g"
  force moment/1(Fb (X Y Z)) -> Gain/1
  force moment/2(M (L M N)) -> Gain1/1
  6DoF (Euler Angles)1/3 -> Bus Creator/3  "Euler"
  Product/1 -> 6DoF (Euler Angles)1/1
  Gain1/1 -> Product1/2
  Product1/1 -> 6DoF (Euler Angles)1/2
  Gain/1 -> Product/2
  Switch2/1 -> Product1/1, Product/1  "是否关闭力输出"
  Fly/1 -> Switch2/1
  SW/1 -> Switch2/2
  init/1 -> Switch2/3
  Flight Conditions/3(amsl) -> Bus Creator/11  "AMSL"
  Flight Conditions/2(lon_deg) -> Bus Creator/10  "lon_deg"
  Flight Conditions/1(lat_deg) -> Bus Creator/9  "lat_deg"
  Flight Conditions/4(Alpha) -> Bus Creator/12  "alpha"
  Flight Conditions/8(EAS) -> Bus Creator/16  "EAS"

== system eVTOL_PX4_2023b/Subsystem1/airframe1 ==
  note: 只进行纵向[1,0,1][0,1,0]
      | 进行纵向+横向[1,1,1][1,1,0]
      | 进行纵向+航向[1,0,1][0,1,1]
  EnvmData : Inport
  prop : Inport  Port=2
  Act_surface : Inport  Port=3
  SW : Inport  Port=4
  6DoF (Euler Angles)1 : aerolibobsolete/6DoF (Euler Angles)  units=Metric (MKS)  mtype=Fixed  rep=Euler Angles  xme_0=InitData.Xe  Vm_0=InitData.Vb  eul_0=InitData.Euler+[0,0,0]/57.3  pm_0=InitData.pqr  mass_0=InitData.mass0  mass_e=0.5  mass_f=2.0  inertia=Mass.Inertial  inertia_e=eye(3)  inertia_f=2*eye(3)  k_quat=1.0
  Bus Creator : BusCreator  Inputs=25
  Constant3 : Constant  Value=mass
  Flight Conditions : Subsystem  AncestorBlock=asbhl20vehicle/Vehicle/Aerodynamic/DerivedConditions
      settings: LibrarySourceBlock=asbhl20vehicle/Vehicle/Aerodynamic/DerivedConditions
  Fly : Constant
  Gain : Gain  Gain=[1,0,1]
  Gain1 : Gain  Gain=[0,1,0]
  Product : Product
  Product1 : Product
  Switch2 : Switch  Criteria=u2 > Threshold  SaturateOnIntegerOverflow=off  InputSameDT=off
  force moment : Subsystem
  init : Constant  Value=0
  UAVData : Outport  VectorParamsAs1DForOutWhenUnconnected=off
  wires:
  prop/1 -> force moment/3(prop)
  6DoF (Euler Angles)1/1 -> Bus Creator/1  "Ve"
  6DoF (Euler Angles)1/2 -> Bus Creator/2  "Xe"
  6DoF (Euler Angles)1/8 -> Bus Creator/8  "Ab"
  6DoF (Euler Angles)1/7 -> Bus Creator/7  "pqr_dot"
  6DoF (Euler Angles)1/6 -> Bus Creator/6  "pqr"
  6DoF (Euler Angles)1/5 -> Bus Creator/5  "Vb"
  Act_surface/1 -> force moment/2(Act_surface)
  Bus Creator/1 -> force moment/1(PlantData), Flight Conditions/2(PlantData), UAVData/1  "UAVData"
  EnvmData/1 -> Flight Conditions/1(EnvmData), force moment/4(EnvmData)
  Flight Conditions/1(Alpha) -> Bus Creator/9  "alpha"
  Flight Conditions/3(Beta) -> Bus Creator/11  "beta"
  Flight Conditions/4(V) -> Bus Creator/12  "Va"
  Flight Conditions/5(pqrWind) -> Bus Creator/13  "pqrWind"
  Flight Conditions/6(Mach) -> Bus Creator/14  "mach"
  Flight Conditions/7(Qbar) -> Bus Creator/15  "Q"
  Flight Conditions/8(gamma) -> Bus Creator/16  "gamma"
  Flight Conditions/2(AlphaDot) -> Bus Creator/10  "alphaDot"
  6DoF (Euler Angles)1/4 -> Bus Creator/4  "DCM_be"
  Constant3/1 -> Bus Creator/21  "mass"
  Flight Conditions/9(chi) -> Bus Creator/17  "chi"
  Flight Conditions/10(Po) -> Bus Creator/18  "Po"
  Flight Conditions/11(To) -> Bus Creator/19  "To"
  Flight Conditions/12(g) -> Bus Creator/20  "g"
  force moment/1(Fb (X Y Z)) -> Gain/1
  force moment/2(M (L M N)) -> Gain1/1
  6DoF (Euler Angles)1/3 -> Bus Creator/3  "Euler"
  Product/1 -> 6DoF (Euler Angles)1/1
  Gain1/1 -> Product1/2
  Product1/1 -> 6DoF (Euler Angles)1/2
  Gain/1 -> Product/2
  Switch2/1 -> Product1/1, Product/1  "是否关闭力输出"
  init/1 -> Switch2/3
  Fly/1 -> Switch2/1
  SW/1 -> Switch2/2
  Flight Conditions/13(lat_deg) -> Bus Creator/22  "lat_deg"
  Flight Conditions/14(lon_deg) -> Bus Creator/23  "lon_deg"
  Flight Conditions/15(amsl) -> Bus Creator/24  "AMSL"
  Flight Conditions/16(EAS) -> Bus Creator/25  "EAS"

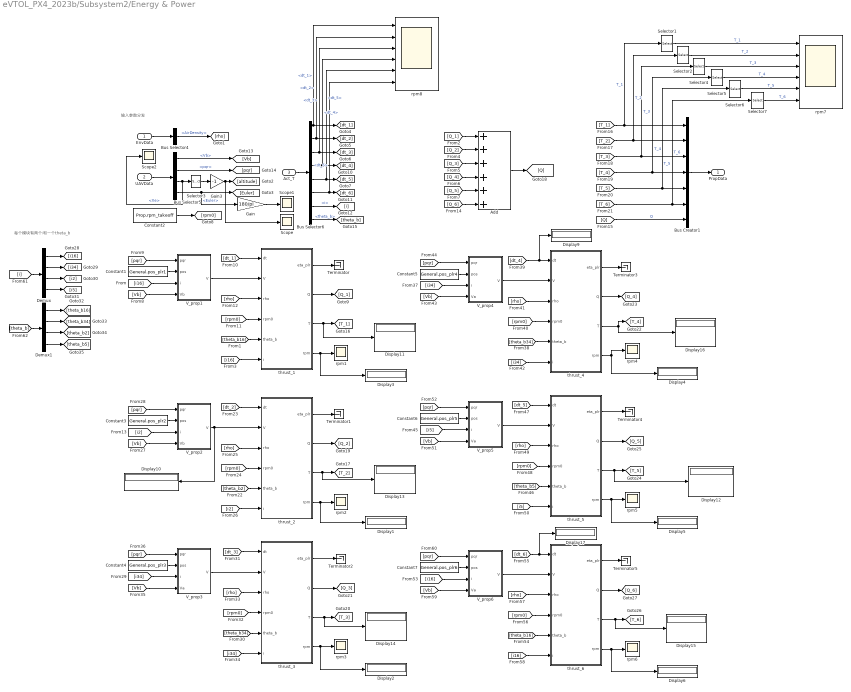
== system eVTOL_PX4_2023b/Subsystem2/Energy & Power ==
  note: 每个模块有两个i和一个theta_b
  note: 输入参数分发
  EnvData : Inport
  UAVData : Inport  Port=2
  Act_T : Inport  Port=3
  Add : Sum  Inputs=++++++
  Bus Creator1 : BusCreator  Inputs=7
  Bus Selector4 : BusSelector  OutputSignals=AirDensity
  Bus Selector5 : BusSelector  OutputSignals=Vb,pqr,Xe,Euler
  Bus Selector6 : BusSelector  OutputSignals=dt_1,dt_2,dt_3,dt_4,dt_5,dt_6,i,theta_b
  Constant1 : Constant  Value=General.pos_plr1
  Constant2 : Constant  Value=Prop.rpm_takeoff
  Constant3 : Constant  Value=General.pos_plr2
  Constant4 : Constant  Value=General.pos_plr3
  Constant5 : Constant  Value=General.pos_plr4
  Constant6 : Constant  Value=General.pos_plr5
  Constant7 : Constant  Value=General.pos_plr6
  Demux : Demux
  Demux1 : Demux
  Display{1..6,9..17} (15 alike) : Display
  Gain : Gain  Gain=180/pi
  Gain3 : Gain  Gain=-1
  Scope : Scope
  Scope1 : Scope
  Scope2 : Scope
  Selector{1..7} (7 alike) : Selector  InputPortWidth=3  IndexOptions=Index vector (dialog)  Indices=3  OutputSizes=1
  Terminator{,1..5} (6 alike) : Terminator
  V_prop1 : Subsystem
  V_prop2 : Subsystem
  V_prop3 : Subsystem
  V_prop4 : Subsystem
  V_prop5 : Subsystem
  V_prop6 : Subsystem
  rpm{1..6} (6 alike) : Scope
  rpm7 : Scope  NumInputPorts=6
  rpm8 : Scope  NumInputPorts=6
  thrust_1 : Subsystem
  thrust_2 : Subsystem
  thrust_3 : Subsystem
  thrust_4 : Subsystem
  thrust_5 : Subsystem
  thrust_6 : Subsystem
  PropData : Outport  VectorParamsAs1DForOutWhenUnconnected=off
  wires:
  Act_T/1 -> Bus Selector6/1
  [dt_1] -> thrust_1/1(dt)
  thrust_1/4(rpm) -> Display3/1, rpm1/1
  Constant1/1 -> V_prop1/2(pos)
  [rho] -> thrust_1/3(rho)
  [rpm0] -> thrust_1/4(rpm0)
  thrust_1/1(eta_plr) -> Terminator/1
  [pqr] -> V_prop1/1(pqr)
  [Vb] -> V_prop1/4(Vb)
  EnvData/1 -> Bus Selector4/1
  Bus Selector4/1 -> [rho]  "<AirDensity>"
  Bus Selector5/2 -> [pqr]  "<pqr>"
  Selector3/1 -> Gain3/1
  UAVData/1 -> Bus Selector5/1
  Bus Selector5/4 -> Gain/1, [Euler]  "<Euler>"
  Bus Selector5/1 -> [Vb]  "<Vb>"
  Bus Selector5/3 -> Scope2/1, Selector3/1  "<Xe>"
  Bus Selector6/1 -> rpm8/1, [dt_1]  "<dt_1>"
  Bus Selector6/5 -> rpm8/5, [dt_5]  "<dt_5>"
  Bus Selector6/3 -> rpm8/3, [dt_3]  "<dt_3>"
  Bus Selector6/2 -> [dt_2], rpm8/2  "<dt_2>"
  V_prop1/1(V) -> thrust_1/2(V)
  [i16] -> V_prop1/3(i)
  Constant2/1 -> [rpm0]
  [theta_b16] -> thrust_1/5(theta_b)
  thrust_1/2(Q) -> [Q_1]
  Bus Selector6/4 -> rpm8/4, [dt_4]  "<dt_4>"
  Bus Selector6/6 -> rpm8/6, [dt_6]  "<dt_6>"
  Bus Selector6/7 -> [i]  "<i>"
  Bus Selector6/8 -> [theta_b]  "<theta_b>"
  [i16] -> thrust_1/6(i)
  thrust_1/3(T) -> Display11/1, [T_1]
  [Q_1] -> Add/1
  [Q_6] -> Add/6
  [Q_5] -> Add/5
  [Q_4] -> Add/4
  [Q_3] -> Add/3
  [Q_2] -> Add/2
  Add/1 -> [Q]
  [Q] -> Bus Creator1/7  "Q"
  [T_1] -> Selector1/1, Bus Creator1/1  "T_1"
  [T_2] -> Selector2/1, Bus Creator1/2  "T_2"
  [T_3] -> Bus Creator1/3, Selector4/1  "T_3"
  [T_4] -> Bus Creator1/4, Selector5/1  "T_4"
  [T_5] -> Bus Creator1/5, Selector6/1  "T_5"
  [T_6] -> Bus Creator1/6, Selector7/1  "T_6"
  Bus Creator1/1 -> PropData/1
  [theta_b2] -> thrust_2/5(theta_b)
  Constant3/1 -> V_prop2/2(pos)
  [dt_2] -> thrust_2/1(dt)
  V_prop2/1(V) -> Display10/1, thrust_2/2(V)
  thrust_2/2(Q) -> [Q_2]
  thrust_2/1(eta_plr) -> Terminator1/1
  [i2] -> V_prop2/3(i)
  thrust_2/3(T) -> [T_2], Display13/1
  [rpm0] -> thrust_2/4(rpm0)
  [Vb] -> V_prop2/4(Vb)
  [pqr] -> V_prop2/1(pqr)
  [i2] -> thrust_2/6(i)
  thrust_2/4(rpm) -> rpm2/1, Display1/1
  [rho] -> thrust_2/3(rho)
  [rho] -> thrust_3/3(rho)
  [pqr] -> V_prop3/1(pqr)
  [Vb] -> V_prop3/4(Va)
  [i34] -> V_prop3/3(i)
  thrust_3/2(Q) -> [Q_3]
  V_prop3/1(V) -> thrust_3/2(V)
  [rpm0] -> thrust_3/4(rpm0)
  [dt_3] -> thrust_3/1(dt)
  thrust_3/4(rpm) -> Display2/1, rpm3/1
  [theta_b34] -> thrust_3/5(theta_b)
  Constant4/1 -> V_prop3/2(pos)
  thrust_3/1(eta_plr) -> Terminator2/1
  [i34] -> thrust_3/6(i)
  thrust_3/3(T) -> Display14/1, [T_3]
  [i34] -> thrust_4/6(i)
  [theta_b34] -> thrust_4/5(theta_b)
  Constant5/1 -> V_prop4/2(pos)
  thrust_4/1(eta_plr) -> Terminator3/1
  thrust_4/3(T) -> [T_4], Display16/1
  [dt_4] -> Display9/1, thrust_4/1(dt)
  V_prop4/1(V) -> thrust_4/2(V)
  [rpm0] -> thrust_4/4(rpm0)
  [i34] -> V_prop4/3(i)
  thrust_4/4(rpm) -> rpm4/1, Display4/1
  [Vb] -> V_prop4/4(Va)
  [pqr] -> V_prop4/1(pqr)
  [rho] -> thrust_4/3(rho)
  thrust_4/2(Q) -> [Q_4]
  thrust_5/2(Q) -> [Q_5]
  thrust_5/3(T) -> Display12/1, [T_5]
  [rho] -> thrust_5/3(rho)
  [pqr] -> V_prop5/1(pqr)
  [rpm0] -> thrust_5/4(rpm0)
  Constant6/1 -> V_prop5/2(pos)
  thrust_5/1(eta_plr) -> Terminator4/1
  [dt_5] -> thrust_5/1(dt)
  thrust_5/4(rpm) -> Display5/1, rpm5/1
  [i5] -> V_prop5/3(i)
  V_prop5/1(V) -> thrust_5/2(V)
  [i5] -> thrust_5/6(i)
  [theta_b5] -> thrust_5/5(theta_b)
  [Vb] -> V_prop5/4(Va)
  [i16] -> V_prop6/3(i)
  [Vb] -> V_prop6/4(Va)
  thrust_6/1(eta_plr) -> Terminator5/1
  V_prop6/1(V) -> thrust_6/2(V)
  [dt_6] -> Display17/1, thrust_6/1(dt)
  [theta_b16] -> thrust_6/5(theta_b)
  thrust_6/2(Q) -> [Q_6]
  thrust_6/3(T) -> Display15/1, [T_6]
  Constant7/1 -> V_prop6/2(pos)
  [rho] -> thrust_6/3(rho)
  thrust_6/4(rpm) -> Display6/1, rpm6/1
  [pqr] -> V_prop6/1(pqr)
  [rpm0] -> thrust_6/4(rpm0)
  [i16] -> thrust_6/6(i)
  Selector1/1 -> rpm7/1  "T_1"
  Selector2/1 -> rpm7/2  "T_2"
  Selector4/1 -> rpm7/3  "T_3"
  Selector5/1 -> rpm7/4  "T_4"
  Selector6/1 -> rpm7/5  "T_5"
  Selector7/1 -> rpm7/6  "T_6"
  Gain3/1 -> Scope/1, [altitude]
  Gain/1 -> Scope1/1
  [i] -> Demux/1
  Demux/1 -> [i16]
  Demux/2 -> [i34]
  Demux/3 -> [i2]
  Demux/4 -> [i5]
  Demux1/2 -> [theta_b34]
  Demux1/3 -> [theta_b2]
  Demux1/1 -> [theta_b16]
  [theta_b] -> Demux1/1
  Demux1/4 -> [theta_b5]

== system eVTOL_PX4_2023b/Subsystem2/Environment ==
  plane : Inport
  Bus Creator : BusCreator  Inputs=8
  Bus Selector : BusSelector  OutputSignals=Xe,Ve,DCM_be
  COESA Atmosphere Model : aerolibatmos2/COESA Atmosphere Model  units=Metric (MKS)  spec=1976 COESA-extended U.S. Standard Atmosphere  model=Profile  profile_var=High temperature  profile_percent=1%  profile_alt=5 km (16404 ft)  envelope_var=High temperature  envelope_percent=1%  action=Warning
  Height : Selector  InputPortWidth=3  IndexOptions=Index vector (dialog)  Indices=[3]  OutputSizes=1
  Latitude : Constant  Value=40
  Terrain : Subsystem
  WGS84 Gravity Model : aerolibobsolete/WGS84 Gravity Model  model=WGS84 Taylor Series  units=Metric (MKS)  no_atmos=on  precessing=on  month=February  day=1  year=2000  no_centrifugal=on  action=None
  Wind Models : Subsystem
  x : Selector  InputPortWidth=3  IndexOptions=Index vector (dialog)  Indices=1  OutputSizes=1
  z-->h : Abs
  Envm : Outport  InitialOutput=0  VectorParamsAs1DForOutWhenUnconnected=off
  wires:
  COESA Atmosphere Model/4 -> Bus Creator/7  "AirDensity"
  COESA Atmosphere Model/2 -> Bus Creator/5  "a"
  COESA Atmosphere Model/3 -> Bus Creator/6  "Po"
  COESA Atmosphere Model/1 -> Bus Creator/4  "To"
  Height/1 -> z-->h/1
  Bus Creator/1 -> Envm/1  "EnvmData"
  plane/1 -> Bus Selector/1
  z-->h/1 -> COESA Atmosphere Model/1, WGS84 Gravity Model/1, Wind Models/3(Altitude)
  Bus Selector/1 -> x/1, Terrain/1(Xe), Height/1  "<Xe>"
  Bus Selector/2 -> Wind Models/2(Ve)  "<Ve>"
  Bus Selector/3 -> Wind Models/4(DCM)  "<DCM_be>"
  Latitude/1 -> WGS84 Gravity Model/2
  WGS84 Gravity Model/1 -> Bus Creator/8  "g"
  Terrain/1(hground) -> Bus Creator/1  "hground"
  Wind Models/1(ug,vg,wg1) -> Bus Creator/2
  Wind Models/2(pg,qg,rg1) -> Bus Creator/3
  x/1 -> Wind Models/1(Xe_x)
